simulink model "model_build"  (R2024b)
settings: Solver=VariableStepAuto  StartTime=0.0  StopTime=100  RelTol=1e-3
libraries: cstblocks x6
settings Model: Creator=Qiyao  LastModifiedBy=Qiyao

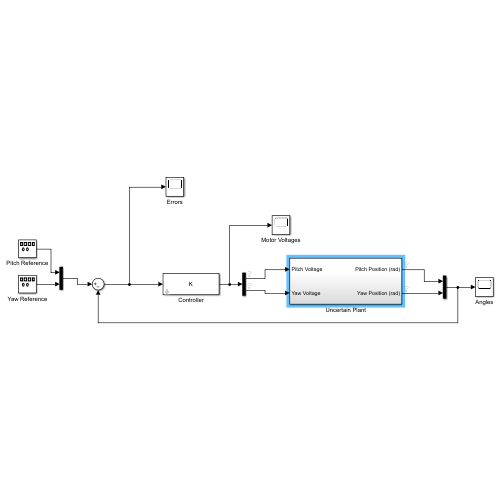
[thumbnail: Simulink's stored preview of the top-level diagram]
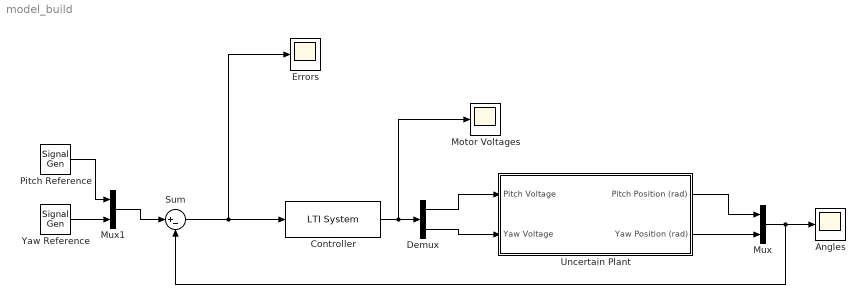
== system model_build ==
  Angles : Scope
  Controller : cstblocks/LTI System  sys=K  IC=[]  PadeOrder=0
  Demux : Demux  Outputs=2
  Errors : Scope
  Motor Voltages : Scope
  Mux : Mux  Inputs=2
  Mux1 : Mux  Inputs=2
  "Pitch Reference " : SignalGenerator  WaveForm=square  Amplitude=pi/6  Frequency=0.02
  Sum : Sum  Inputs=|+-
  Uncertain Plant : Subsystem
  Yaw Reference : SignalGenerator  WaveForm=square  Amplitude=pi/4  Frequency=0.02
  wires:
  Uncertain Plant/2(Yaw Position (rad)) -> Mux/2
  Controller/1 -> Motor Voltages/1, Demux/1
  Sum/1 -> Errors/1, Controller/1
  Uncertain Plant/1(Pitch Position (rad)) -> Mux/1
  Mux1/1 -> Sum/1
  Mux/1 -> Sum/2, Angles/1
  Demux/2 -> Uncertain Plant/2(Yaw Voltage)
  Yaw Reference/1 -> Mux1/2
  Demux/1 -> Uncertain Plant/1(Pitch Voltage)
  "Pitch Reference "/1 -> Mux1/1

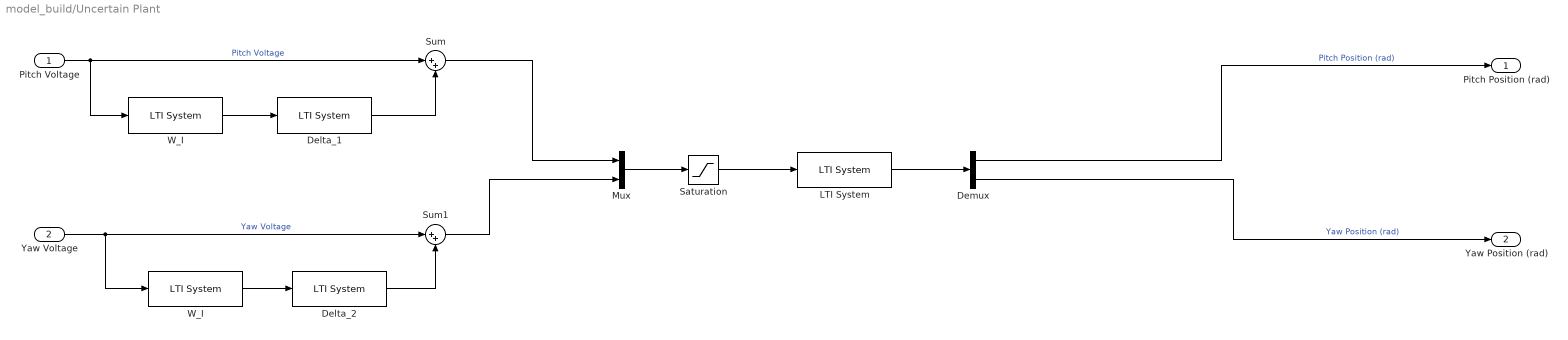
== system model_build/Uncertain Plant ==
  Pitch Voltage : Inport
  Yaw Voltage : Inport  Port=2
  Delta_1 : cstblocks/LTI System  sys=Delta_1  IC=[]  PadeOrder=0
  Delta_2 : cstblocks/LTI System  sys=Delta_2  IC=[]  PadeOrder=0
  Demux : Demux  Outputs=2
  LTI System : cstblocks/LTI System  sys=G_nominal  IC=[]  PadeOrder=0
  Mux : Mux  Inputs=2
  Saturation : Saturate  UpperLimit=25  LowerLimit=-25
  Sum : Sum  Inputs=|++
  Sum1 : Sum  Inputs=|++
  W_I : cstblocks/LTI System  sys=W_I_Pitch  IC=[]  PadeOrder=0
  "W_I " : cstblocks/LTI System  sys=W_I_Yaw  IC=[]  PadeOrder=0
  Pitch Position (rad) : Outport
  Yaw Position (rad) : Outport  Port=2
  wires:
  W_I/1 -> Delta_1/1
  Pitch Voltage/1 -> W_I/1, Sum/1  "Pitch Voltage"
  Delta_1/1 -> Sum/2
  Yaw Voltage/1 -> "W_I "/1, Sum1/1  "Yaw Voltage"
  Delta_2/1 -> Sum1/2
  "W_I "/1 -> Delta_2/1
  Sum/1 -> Mux/1
  Sum1/1 -> Mux/2
  LTI System/1 -> Demux/1
  Demux/1 -> Pitch Position (rad)/1  "Pitch Position (rad)"
  Demux/2 -> Yaw Position (rad)/1  "Yaw Position (rad)"
  Mux/1 -> Saturation/1
  Saturation/1 -> LTI System/1
